simulink model "PhantomX_MK4"  (R2023a)
settings: Solver=FixedStepAuto  StartTime=0.0  StopTime=inf  FixedStep=0.00005  RelTol=1e-3
values from neighbouring files (symbols this model uses):
  angle_offsets_LF_RB = [45, 14.03624347, 60.58440117]    [InitialisationScript.m]    (also in simulation_setup.m)
  angle_offsets_middle = [0, 14.03624347, 60.58440117]    [InitialisationScript.m]    (also in simulation_setup.m)
  angle_offsets_RF_LB = [-45, 14.03624347, 60.58440117]    [InitialisationScript.m]    (also in simulation_setup.m)
  N = 16    [rl_setup.m]
  pid_D = 1    [InitialisationScript.m]    (also in simulation_setup.m)
  pid_filter_N = 100    [InitialisationScript.m]    (also in simulation_setup.m = 1000)
  pid_I = 0.2    [InitialisationScript.m]    (also in simulation_setup.m = 0.1)
  pid_P = 3    [InitialisationScript.m]    (also in simulation_setup.m = 600)
  x_offset = 0.2    [InitialisationScript.m]
  z_offset = -0.14    [InitialisationScript.m]
undefined symbols (not defined in the file or in its folder): LBL_sensory_data, left_side_torques, LFL_sensory_data, LML_sensory_data, RBL_sensory_data, RFL_sensory_data, right_side_torques, RML_sensory_data, X, Y, Z
libraries: sm_lib x30, slpidlib x18, Custom_Library x13, robotmaniplib x6, nesl_utility x3, rllib x1, simulink_extras x1
(part 1 of 4)
settings Model: SimulationMode=accelerator  PacingRate=0.089000  Creator=basti  LastModifiedBy=basti
settings SolverCC: EnableFixedStepZeroCrossing=on
settings ExplorerConfigSet: InternalSimMechanicsExplorerSettings="<ExplorerConfiguration><canonicalview>default</canonicalview><AnimationSetting><BasePlaybackSpeed>1.0</BasePlaybackSpeed><PlaybackSpeedFactor>1.0</PlaybackSpeedFactor></AnimationSetting><TilePanel><TileInfo><Tiles Columns=\"1\" Count=\"1\" Rows=\"1\"><Column Weight=\"1\"/><Row Weight=\"1\"/><Tile Height=\"1\" Width=\"1\" X=\"0\" Y=\"0\"/></Tiles></TileInfo><SceneInfo><SceneViewer><BGColor><R>0.800000011920928955</R><G>0.800000011920928955</G><B>0.800000011920928955</B></BGColor><Camera><DoPerspective>off</DoPerspective><Position><X>0.0139405011924200652</X><Y>-25.6990972548707113</Y><Z>0.0237848079060223108</Z></Position><Center><X>0.0139405011924200652</X><Y>8.89140117983633349e-07</Y><Z>0.0237848079060223108</Z></Center><Up><X>0</X><Y>-0</Y><Z>1</Z></Up><ViewLimDist>1</ViewLimDist><YLim>0.273259206556581868</YLim><XLim>0.411669828872019972</XLim></Camera></SceneViewer></SceneInfo></TilePanel><MechEditorPanel><Cameras/><GfxPanelCameraMap/><VideoCreator><PlaybackSpeedRatio>1.0</PlaybackSpeedRatio><FrameRate>60</FrameRate><VideoFormat>MPEG-4</VideoFormat><FrameSize>[1920 1080]</FrameSize></VideoCreator></MechEditorPanel></ExplorerConfiguration>"

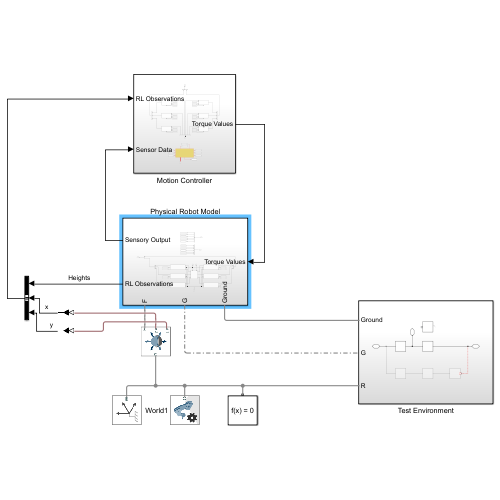
[thumbnail: Simulink's stored preview of the top-level diagram]
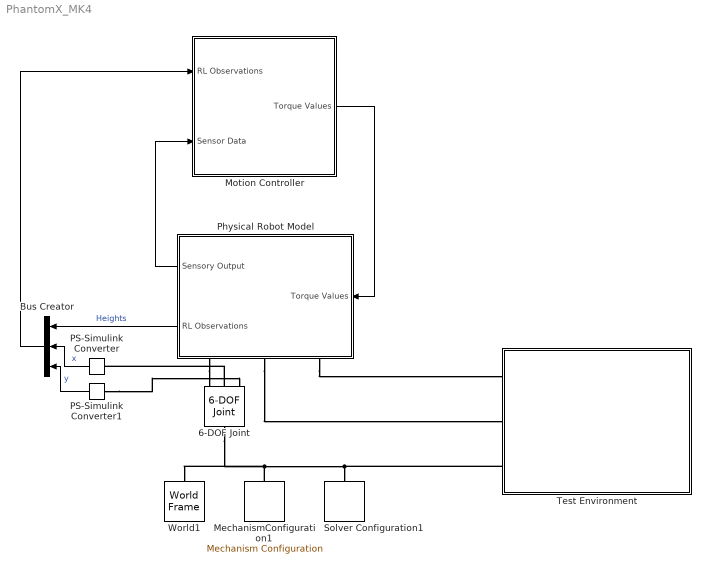
== system PhantomX_MK4 ==
  6-DOF Joint : sm_lib/Joints/6-DOF Joint  JointMode=Normal  SenseConstraintForce=off  SenseConstraintForceX=off  SenseConstraintForceY=off  SenseConstraintForceZ=off  SenseConstraintTorque=off  SenseConstraintTorqueX=off  SenseConstraintTorqueY=off  SenseConstraintTorqueZ=off  SenseTotalForce=off  SenseTotalForceX=off  SenseTotalForceY=off  SenseTotalForceZ=off  SenseTotalTorque=off  SenseTotalTorqueX=off  SenseTotalTorqueY=off  SenseTotalTorqueZ=off  CompositeWrenchDir=FollowerOnBase  CompositeWrenchFrame=BaseFrame  PxEquilibriumPosition=0  PxEquilibriumPositionUnits=m  PxSpringStiffness=0  PxSpringStiffnessUnits=N/m  PxDampingCoefficient=1e-8  PxDampingCoefficientUnits=N/(m/s)  PxTorqueActuationMode=NoTorque  PxMotionActuationMode=ComputedMotion  PxSensePosition=on  PxSenseVelocity=off  PxSenseAcceleration=off  PxSenseTorqueForce=off  PxSenseLowerLimitTorqueForce=off  PxSenseUpperLimitTorqueForce=off  PxLowerLimitSpecify=off  PxLowerLimitBound=-1  PxLowerLimitBoundUnits=m  PxLowerLimitStiffness=1e6  PxLowerLimitStiffnessUnits=N/m  PxLowerLimitDamping=1e3  PxLowerLimitDampingUnits=N/(m/s)  PxLowerLimitTransitionRegionWidth=1e-4  PxLowerLimitTransitionRegionWidthUnits=m  PxUpperLimitSpecify=off  PxUpperLimitBound=1  PxUpperLimitBoundUnits=m  PxUpperLimitStiffness=1e6  PxUpperLimitStiffnessUnits=N/m  PxUpperLimitDamping=1e3  PxUpperLimitDampingUnits=N/(m/s)  PxUpperLimitTransitionRegionWidth=1e-4  PxUpperLimitTransitionRegionWidthUnits=m  PxPositionTargetSpecify=off  PxPositionTargetPriority=High  PxPositionTargetValue=0  PxPositionTargetValueUnits=m  PxVelocityTargetSpecify=off  PxVelocityTargetPriority=High  PxVelocityTargetValue=0  PxVelocityTargetValueUnits=m/s  PyEquilibriumPosition=0  PyEquilibriumPositionUnits=m  PySpringStiffness=0  PySpringStiffnessUnits=N/m  PyDampingCoefficient=1e-8  PyDampingCoefficientUnits=N/(m/s)  PyTorqueActuationMode=NoTorque  PyMotionActuationMode=ComputedMotion  PySensePosition=on  PySenseVelocity=off  PySenseAcceleration=off  PySenseTorqueForce=off  PySenseLowerLimitTorqueForce=off  PySenseUpperLimitTorqueForce=off  PyLowerLimitSpecify=off  PyLowerLimitBound=-1  PyLowerLimitBoundUnits=m  PyLowerLimitStiffness=1e6  PyLowerLimitStiffnessUnits=N/m  PyLowerLimitDamping=1e3  PyLowerLimitDampingUnits=N/(m/s)  PyLowerLimitTransitionRegionWidth=1e-4  PyLowerLimitTransitionRegionWidthUnits=m  PyUpperLimitSpecify=off  PyUpperLimitBound=1  PyUpperLimitBoundUnits=m  PyUpperLimitStiffness=1e6  PyUpperLimitStiffnessUnits=N/m  PyUpperLimitDamping=1e3  PyUpperLimitDampingUnits=N/(m/s)  PyUpperLimitTransitionRegionWidth=1e-4  PyUpperLimitTransitionRegionWidthUnits=m  PyPositionTargetSpecify=off  PyPositionTargetPriority=High  PyPositionTargetValue=0  PyPositionTargetValueUnits=m  PyVelocityTargetSpecify=off  PyVelocityTargetPriority=High  PyVelocityTargetValue=0  PyVelocityTargetValueUnits=m/s  PzEquilibriumPosition=0  PzEquilibriumPositionUnits=m  PzSpringStiffness=0  PzSpringStiffnessUnits=N/m  PzDampingCoefficient=1e-8  PzDampingCoefficientUnits=N/(m/s)  PzTorqueActuationMode=NoTorque  PzMotionActuationMode=ComputedMotion  PzSensePosition=off  PzSenseVelocity=off  PzSenseAcceleration=off  PzSenseTorqueForce=off  PzSenseLowerLimitTorqueForce=off  PzSenseUpperLimitTorqueForce=off  PzLowerLimitSpecify=off  PzLowerLimitBound=-1  PzLowerLimitBoundUnits=m  PzLowerLimitStiffness=1e6  PzLowerLimitStiffnessUnits=N/m  PzLowerLimitDamping=1e3  PzLowerLimitDampingUnits=N/(m/s)  PzLowerLimitTransitionRegionWidth=1e-4  PzLowerLimitTransitionRegionWidthUnits=m  PzUpperLimitSpecify=off  PzUpperLimitBound=1  PzUpperLimitBoundUnits=m  PzUpperLimitStiffness=1e6  PzUpperLimitStiffnessUnits=N/m  PzUpperLimitDamping=1e3  PzUpperLimitDampingUnits=N/(m/s)  PzUpperLimitTransitionRegionWidth=1e-4  PzUpperLimitTransitionRegionWidthUnits=m  PzPositionTargetSpecify=off  PzPositionTargetPriority=High  PzPositionTargetValue=0  PzPositionTargetValueUnits=m  PzVelocityTargetSpecify=off  PzVelocityTargetPriority=High  PzVelocityTargetValue=0  PzVelocityTargetValueUnits=m/s  SphEqPosRotationMethod=None  SphEqPosRotationAngleUnits=deg  SphEqPosRotationStandardAxis=+Z  SphEqPosRotationAngle=0.0  SphEqPosRotationArbitraryAxis=[0 0 1]  SphEqPosFollAlignAxisA=+X  SphEqPosBaseAlignAxisA=+Y  SphEqPosFollAlignAxisB=+Y  SphEqPosBaseAlignAxisB=+Z  SphEqPosRotationSequenceAxes=FollowerAxes  SphEqPosRotationSequence=XYX  SphEqPosRotationSequenceAngles=[0 0 0]  SphEqPosRotationSequenceAnglesUnits=deg  SphEqPosRotationMatrix=[1 0 0; 0 1 0; 0 0 1]  SphEqPosQuaternion=[1 0 0 0]  SphSpringStiffness=0  SphSpringStiffnessUnits=N*m/deg  SphDampingCoefficient=0  SphDampingCoefficientUnits=N*m/(deg/s)  SphActuateTorqueX=off  SphActuateTorqueY=off  SphActuateTorqueZ=off  SphActuateTorque=off  SphTorqueActuationMode=NoTorque  SphMotionActuationMode=ComputedMotion  SphActuationFrame=BaseFrame  SphSensePosition=off  SphSenseVelocityX=off  SphSenseVelocityY=off  SphSenseVelocityZ=off  SphSenseVelocity=off  SphSenseAccelerationX=off  SphSenseAccelerationY=off  SphSenseAccelerationZ=off  SphSenseAcceleration=off  SphSenseTorqueX=off  SphSenseTorqueY=off  SphSenseTorqueZ=off  SphSenseTorqueForce=off  SphSenseLowerLimitTorqueMag=off  SphSenseUpperLimitTorqueMag=off  SphSensingFrame=BaseFrame  SphLowerLimitSpecify=off  SphLowerLimitBound=15  SphLowerLimitBoundUnits=deg  SphLowerLimitStiffness=1e4  SphLowerLimitStiffnessUnits=N*m/deg  SphLowerLimitDamping=10  SphLowerLimitDampingUnits=N*m/(deg/s)  SphLowerLimitTransitionRegionWidth=0.1  SphLowerLimitTransitionRegionWidthUnits=deg  SphUpperLimitSpecify=off  SphUpperLimitBound=45  SphUpperLimitBoundUnits=deg  SphUpperLimitStiffness=1e4  SphUpperLimitStiffnessUnits=N*m/deg  SphUpperLimitDamping=10  SphUpperLimitDampingUnits=N*m/(deg/s)  SphUpperLimitTransitionRegionWidth=0.1  SphUpperLimitTransitionRegionWidthUnits=deg  SphPositionTargetRotationMethod=None  SphPositionTargetRotationAngleUnits=deg  SphPositionTargetRotationStandardAxis=+Z  SphPositionTargetRotationAngle=0.0  SphPositionTargetRotationArbitraryAxis=[0 0 1]  SphPositionTargetFollAlignAxisA=+X  SphPositionTargetBaseAlignAxisA=+Y  SphPositionTargetFollAlignAxisB=+Y  SphPositionTargetBaseAlignAxisB=+Z  SphPositionTargetRotationSequenceAxes=FollowerAxes  SphPositionTargetRotationSequence=XYX  SphPositionTargetRotationSequenceAngles=[0 0 0]  SphPositionTargetRotationSequenceAnglesUnits=deg  SphPositionTargetRotationMatrix=[1 0 0; 0 1 0; 0 0 1]  SphPositionTargetQuaternion=[1 0 0 0]  SphPositionTargetSpecify=off  SphPositionTargetPriority=High  SphVelocityTargetValue=[0 0 0]  SphVelocityTargetValueUnits=deg/s  SphVelocityTargetSpecify=off  SphVelocityTargetPriority=High  SphVelocityTargetInFollowerFrame=on
  Bus Creator : BusCreator  Inputs=3
  MechanismConfiguration1 : sm_lib/Utilities/Mechanism Configuration  UniformGravity=Constant  GravityVector=gravity_vector  GravityVectorUnits=m/s^2  LinearizationDelta=1e-4  JointModeTransitionNonlinearIterations=4
  Motion Controller : Subsystem
  PS-Simulink Converter : nesl_utility/PS-Simulink Converter  PhysicalDomain=network_engine_domain  SubClassName=ps_output  LeftPortType=input  RightPortType=output  PseudoPeriodic=off  Frequencies=[]  VectorFormat=inherit  Unit=inherit  AffineConversion=off
  PS-Simulink Converter1 : nesl_utility/PS-Simulink Converter  PhysicalDomain=network_engine_domain  SubClassName=ps_output  LeftPortType=input  RightPortType=output  PseudoPeriodic=off  Frequencies=[]  VectorFormat=inherit  Unit=inherit  AffineConversion=off
  Physical Robot Model : Subsystem
      settings: PortSchema="{\"entries\":[{\"content\":{\"sides\":[{\"content\":{\"connectorIds\":[\"In1\"]},\"type\":\"ConnectorPlacement.EquallySpacedRectSide\",\"uuid\":\"88f2b8a6-de04-409c-a7b8-092446ee7a8a\"},{\"content\":{\"connectorIds\":[\"Out1\",\"Out2\"],\"side\":\"RIGHT\"},\"type\":\"ConnectorPlacement.EquallySpacedRectSide\",\"uuid\":\"05452a16-e9b5-441f-b64c-cc8b5f8bc9a9\"},{\"content\":{\"side\":\"TOP\"},\"type\":\"ConnectorPlacement.EquallySpacedRectSide\",\"uuid\":\"4b1c2960-246e-4fa9-be3c-7b063d456f3b\"},{\"content\":{\"connectorIds\":[\"RConn1\",\"RConn2\",\"RConn3\"],\"side\":\"BOTTOM\"},\"type\":\"ConnectorPlacement.EquallySpacedRectSide\",\"uuid\":\"877efe3a-863b-4f41-9fff-16e3adccfccc\"}]},\"type\":\"ConnectorPlacement.EquallySpacedConnector\",\"uuid\":\"79d07eaf-febf-441f-a139-eb85057738c3\"}],\"packageUris\":[\"http://schema.mathworks.com/mf0/Connector/R2020b\"],\"version\":\"1.0\"}"
  Solver Configuration1 : nesl_utility/Solver Configuration  PhysicalDomain=network_engine_domain  SubClassName=solver  LeftPortType=input  RightPortType=generic  Tones=[]  Harmonics=[]  SimulateNoise=off  Profile=off  UseLocalSampling=off  EnableSwitchedLinearOptims=on  FrequencyDomain=off  UseCCode=off  RelTol=0.001  AbsTol=0.001  MinStep=1e-09  ToWorkspace=off  RevertToSquareIcSolve=off  NumHomotopyIterations=100  PhasorMode=off  PhasorModeNumHarmonics=1  ConsistencySolver=NEWTON_XTOL_AFTER_FTOL  IndexReductionMethod=DerivativeReplacement  DoDC=off  ResidualTolerance=1e-09  ConsistencyTolSource=GLOBAL  ConsistencyAbsTol=0.001  ConsistencyRelTol=0.001  ConsistencyTolFactor=1e-4  UseLocalSolver=off  LocalSolverChoice=NE_BACKWARD_EULER_ADVANCER  ResolveIndetEquations=on  FunctionEvalNumThread=1  LocalSolverSampleTime=0.001  DoFixedCost=off  MaxNonlinIter=3  MaxModeIter=2  ComputeImpulses=off  ImpulseIterations=2  LinearAlgebra=Full  LinearAlgebraNumThread=0  EquationFormulation=NE_TIME_EF  DelaysMemoryBudget=2048  AutomaticFiltering=on  FilteringTimeConstant=0.001  PartitionStorageMethod=AS_NEEDED  PartitionMemoryBudget=1024  PartitionMethod=ROBUST
  Test Environment : Subsystem
  World1 : sm_lib/Frames and Transforms/World Frame
  wires:
  Physical Robot Model/1(Sensory Output) -> Motion Controller/2(Sensor Data)
  Motion Controller/1(Torque Values) -> Physical Robot Model/1(Torque Values)
  PS-Simulink Converter/1 -> Bus Creator/2  "x"
  Physical Robot Model/2(RL Observations) -> Bus Creator/1  "Heights"
  Bus Creator/1 -> Motion Controller/1(RL Observations)
  PS-Simulink Converter1/1 -> Bus Creator/3  "y"
  connections:
  MechanismConfiguration1/RConn1 -- World1/RConn1 -- 6-DOF Joint/LConn1 -- Test Environment/LConn3 -- Solver Configuration1/RConn1
  Physical Robot Model/RConn2 -- Test Environment/LConn2
  Physical Robot Model/RConn3 -- 6-DOF Joint/RConn1
  Physical Robot Model/RConn1 -- Test Environment/LConn1
  6-DOF Joint/RConn2 -- PS-Simulink Converter/LConn1
  PS-Simulink Converter1/LConn1 -- 6-DOF Joint/RConn3

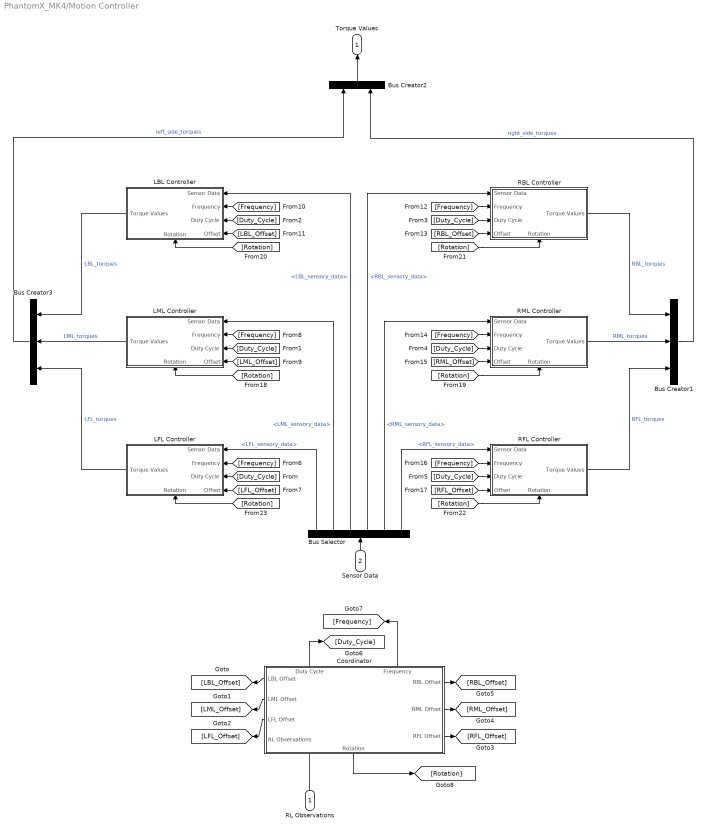
== system PhantomX_MK4/Motion Controller ==
  RL Observations : Inport
  Sensor Data : Inport  Port=2
  Bus Creator1 : BusCreator  Inputs=3
  Bus Creator2 : BusCreator  Inputs=left_side_torques,right_side_torques
  Bus Creator3 : BusCreator  Inputs=3
  Bus Selector : BusSelector  OutputSignals=LFL_sensory_data,LML_sensory_data,LBL_sensory_data,RBL_sensory_data,RML_sensory_data,RFL_sensory_data
  Coordinator : Subsystem
      settings: PortSchema="{\"entries\":[{\"content\":{\"sides\":[{\"content\":{\"connectorIds\":[\"Out7\",\"Out8\",\"Out9\",\"In1\"]},\"type\":\"ConnectorPlacement.EquallySpacedRectSide\",\"uuid\":\"0589587c-a667-4b39-9acd-4e49c48a2b81\"},{\"content\":{\"connectorIds\":[\"Out1\",\"Out2\",\"Out3\"],\"side\":\"RIGHT\"},\"type\":\"ConnectorPlacement.EquallySpacedRectSide\",\"uuid\":\"38142eef-ff42-4a7a-ad69-e4b368cabc10\"},{\"content\":{\"connectorIds\":[\"Out5\",\"Out6\"],\"side\":\"TOP\"},\"type\":\"ConnectorPlacement.EquallySpacedRectSide\",\"uuid\":\"0cab318c-da30-4070-96db-6d2791547378\"},{\"content\":{\"connectorIds\":[\"Out4\"],\"side\":\"BOTTOM\"},\"type\":\"ConnectorPlacement.EquallySpacedRectSide\",\"uuid\":\"5a744909-6628-4943-920b-0f55011947f4\"}]},\"type\":\"ConnectorPlacement.EquallySpacedConnector\",\"uuid\":\"f4523b82-4d9f-456b-8594-48e9d89b7aea\"}],\"packageUris\":[\"http://schema.mathworks.com/mf0/Connector/R2020b\"],\"version\":\"1.0\"}"
  LBL Controller : Subsystem
      settings: PortSchema="{\"entries\":[{\"content\":{\"sides\":[{\"content\":{\"connectorIds\":[\"In1\",\"In2\",\"In3\",\"In4\"]},\"type\":\"ConnectorPlacement.EquallySpacedRectSide\",\"uuid\":\"61807659-790a-4fcc-8eea-bb1747959d2c\"},{\"content\":{\"connectorIds\":[\"Out1\"],\"side\":\"RIGHT\"},\"type\":\"ConnectorPlacement.EquallySpacedRectSide\",\"uuid\":\"beab48f8-df50-4720-a4fe-1084d91255e1\"},{\"content\":{\"side\":\"TOP\"},\"type\":\"ConnectorPlacement.EquallySpacedRectSide\",\"uuid\":\"df2f0e11-b286-4413-8948-937711258f59\"},{\"content\":{\"connectorIds\":[\"In5\"],\"side\":\"BOTTOM\"},\"type\":\"ConnectorPlacement.EquallySpacedRectSide\",\"uuid\":\"177fd513-fdd6-4ae0-8805-86acc5cb073f\"}]},\"type\":\"ConnectorPlacement.EquallySpacedConnector\",\"uuid\":\"735c34ff-c8fb-4d96-b4d8-f985913f524f\"}],\"packageUris\":[\"http://schema.mathworks.com/mf0/Connector/R2020b\"],\"version\":\"1.0\"}"
  LFL Controller : Subsystem
      settings: PortSchema="{\"entries\":[{\"content\":{\"sides\":[{\"content\":{\"connectorIds\":[\"In1\",\"In2\",\"In3\",\"In4\"]},\"type\":\"ConnectorPlacement.EquallySpacedRectSide\",\"uuid\":\"61807659-790a-4fcc-8eea-bb1747959d2c\"},{\"content\":{\"connectorIds\":[\"Out1\"],\"side\":\"RIGHT\"},\"type\":\"ConnectorPlacement.EquallySpacedRectSide\",\"uuid\":\"beab48f8-df50-4720-a4fe-1084d91255e1\"},{\"content\":{\"side\":\"TOP\"},\"type\":\"ConnectorPlacement.EquallySpacedRectSide\",\"uuid\":\"df2f0e11-b286-4413-8948-937711258f59\"},{\"content\":{\"connectorIds\":[\"In5\"],\"side\":\"BOTTOM\"},\"type\":\"ConnectorPlacement.EquallySpacedRectSide\",\"uuid\":\"f745b799-b20b-4ee3-af3a-7f9c6b228ef2\"}]},\"type\":\"ConnectorPlacement.EquallySpacedConnector\",\"uuid\":\"735c34ff-c8fb-4d96-b4d8-f985913f524f\"}],\"packageUris\":[\"http://schema.mathworks.com/mf0/Connector/R2020b\"],\"version\":\"1.0\"}"
  LML Controller : Subsystem
      settings: PortSchema="{\"entries\":[{\"content\":{\"sides\":[{\"content\":{\"connectorIds\":[\"In1\",\"In2\",\"In3\",\"In4\"]},\"type\":\"ConnectorPlacement.EquallySpacedRectSide\",\"uuid\":\"61807659-790a-4fcc-8eea-bb1747959d2c\"},{\"content\":{\"connectorIds\":[\"Out1\"],\"side\":\"RIGHT\"},\"type\":\"ConnectorPlacement.EquallySpacedRectSide\",\"uuid\":\"beab48f8-df50-4720-a4fe-1084d91255e1\"},{\"content\":{\"side\":\"TOP\"},\"type\":\"ConnectorPlacement.EquallySpacedRectSide\",\"uuid\":\"df2f0e11-b286-4413-8948-937711258f59\"},{\"content\":{\"connectorIds\":[\"In5\"],\"side\":\"BOTTOM\"},\"type\":\"ConnectorPlacement.EquallySpacedRectSide\",\"uuid\":\"b53235e4-d895-4a2a-8595-c01fb6c9295f\"}]},\"type\":\"ConnectorPlacement.EquallySpacedConnector\",\"uuid\":\"735c34ff-c8fb-4d96-b4d8-f985913f524f\"}],\"packageUris\":[\"http://schema.mathworks.com/mf0/Connector/R2020b\"],\"version\":\"1.0\"}"
  RBL Controller : Subsystem
      settings: PortSchema="{\"entries\":[{\"content\":{\"sides\":[{\"content\":{\"connectorIds\":[\"In1\",\"In2\",\"In3\",\"In4\"]},\"type\":\"ConnectorPlacement.EquallySpacedRectSide\",\"uuid\":\"61807659-790a-4fcc-8eea-bb1747959d2c\"},{\"content\":{\"connectorIds\":[\"Out1\"],\"side\":\"RIGHT\"},\"type\":\"ConnectorPlacement.EquallySpacedRectSide\",\"uuid\":\"beab48f8-df50-4720-a4fe-1084d91255e1\"},{\"content\":{\"side\":\"TOP\"},\"type\":\"ConnectorPlacement.EquallySpacedRectSide\",\"uuid\":\"df2f0e11-b286-4413-8948-937711258f59\"},{\"content\":{\"connectorIds\":[\"In5\"],\"side\":\"BOTTOM\"},\"type\":\"ConnectorPlacement.EquallySpacedRectSide\",\"uuid\":\"541f6a39-2cd2-4849-82a6-ba8e08840f40\"}]},\"type\":\"ConnectorPlacement.EquallySpacedConnector\",\"uuid\":\"735c34ff-c8fb-4d96-b4d8-f985913f524f\"}],\"packageUris\":[\"http://schema.mathworks.com/mf0/Connector/R2020b\"],\"version\":\"1.0\"}"
  RFL Controller : Subsystem
      settings: PortSchema="{\"entries\":[{\"content\":{\"sides\":[{\"content\":{\"connectorIds\":[\"In1\",\"In2\",\"In3\",\"In4\"]},\"type\":\"ConnectorPlacement.EquallySpacedRectSide\",\"uuid\":\"e919d3cb-cb22-4ae7-9921-75070e82dfc0\"},{\"content\":{\"connectorIds\":[\"Out1\"],\"side\":\"RIGHT\"},\"type\":\"ConnectorPlacement.EquallySpacedRectSide\",\"uuid\":\"1bac186a-4e1d-4bd0-8d36-9d7d141f01e6\"},{\"content\":{\"side\":\"TOP\"},\"type\":\"ConnectorPlacement.EquallySpacedRectSide\",\"uuid\":\"779ab6f5-6e15-4076-9acb-2bf4234ddf49\"},{\"content\":{\"connectorIds\":[\"In5\"],\"side\":\"BOTTOM\"},\"type\":\"ConnectorPlacement.EquallySpacedRectSide\",\"uuid\":\"a3aab620-5d97-425b-8a2a-088ff14d55a6\"}]},\"type\":\"ConnectorPlacement.EquallySpacedConnector\",\"uuid\":\"b8d6bd7a-da61-4133-9438-dd2459d5cc9a\"}],\"packageUris\":[\"http://schema.mathworks.com/mf0/Connector/R2020b\"],\"version\":\"1.0\"}"
  RML Controller : Subsystem
      settings: PortSchema="{\"entries\":[{\"content\":{\"sides\":[{\"content\":{\"connectorIds\":[\"In1\",\"In2\",\"In3\",\"In4\"]},\"type\":\"ConnectorPlacement.EquallySpacedRectSide\",\"uuid\":\"61807659-790a-4fcc-8eea-bb1747959d2c\"},{\"content\":{\"connectorIds\":[\"Out1\"],\"side\":\"RIGHT\"},\"type\":\"ConnectorPlacement.EquallySpacedRectSide\",\"uuid\":\"beab48f8-df50-4720-a4fe-1084d91255e1\"},{\"content\":{\"side\":\"TOP\"},\"type\":\"ConnectorPlacement.EquallySpacedRectSide\",\"uuid\":\"df2f0e11-b286-4413-8948-937711258f59\"},{\"content\":{\"connectorIds\":[\"In5\"],\"side\":\"BOTTOM\"},\"type\":\"ConnectorPlacement.EquallySpacedRectSide\",\"uuid\":\"7df11b11-4116-490c-abf6-aeb9f4bc13f8\"}]},\"type\":\"ConnectorPlacement.EquallySpacedConnector\",\"uuid\":\"735c34ff-c8fb-4d96-b4d8-f985913f524f\"}],\"packageUris\":[\"http://schema.mathworks.com/mf0/Connector/R2020b\"],\"version\":\"1.0\"}"
  Torque Values : Outport
  wires:
  Sensor Data/1 -> Bus Selector/1
  Bus Creator2/1 -> Torque Values/1
  Bus Creator1/1 -> Bus Creator2/2  "right_side_torques"
  Bus Creator3/1 -> Bus Creator2/1  "left_side_torques"
  LFL Controller/1(Torque Values) -> Bus Creator3/3  "LFL_torques"
  LML Controller/1(Torque Values) -> Bus Creator3/2  "LML_torques"
  LBL Controller/1(Torque Values) -> Bus Creator3/1  "LBL_torques"
  RBL Controller/1(Torque Values) -> Bus Creator1/1  "RBL_torques"
  RML Controller/1(Torque Values) -> Bus Creator1/2  "RML_torques"
  RFL Controller/1(Torque Values) -> Bus Creator1/3  "RFL_torques"
  Coordinator/7(LBL Offset) -> [LBL_Offset]
  Coordinator/8(LML Offset) -> [LML_Offset]
  Coordinator/9(LFL Offset) -> [LFL_Offset]
  Coordinator/3(RFL Offset) -> [RFL_Offset]
  Coordinator/2(RML Offset) -> [RML_Offset]
  Coordinator/1(RBL Offset) -> [RBL_Offset]
  Coordinator/5(Duty Cycle) -> [Duty_Cycle]
  Coordinator/6(Frequency) -> [Frequency]
  [Duty_Cycle] -> LFL Controller/3(Duty Cycle)
  [Duty_Cycle] -> LML Controller/3(Duty Cycle)
  [Duty_Cycle] -> LBL Controller/3(Duty Cycle)
  [Duty_Cycle] -> RBL Controller/3(Duty Cycle)
  [Duty_Cycle] -> RML Controller/3(Duty Cycle)
  [Duty_Cycle] -> RFL Controller/3(Duty Cycle)
  [Frequency] -> LFL Controller/2(Frequency)
  [LFL_Offset] -> LFL Controller/4(Offset)
  [LML_Offset] -> LML Controller/4(Offset)
  [Frequency] -> LML Controller/2(Frequency)
  [LBL_Offset] -> LBL Controller/4(Offset)
  [Frequency] -> LBL Controller/2(Frequency)
  [Frequency] -> RBL Controller/2(Frequency)
  [RBL_Offset] -> RBL Controller/4(Offset)
  [RML_Offset] -> RML Controller/4(Offset)
  [Frequency] -> RML Controller/2(Frequency)
  [Frequency] -> RFL Controller/2(Frequency)
  [RFL_Offset] -> RFL Controller/4(Offset)
  Bus Selector/4 -> RBL Controller/1(Sensor Data)  "<RBL_sensory_data>"
  Bus Selector/1 -> LFL Controller/1(Sensor Data)  "<LFL_sensory_data>"
  Bus Selector/2 -> LML Controller/1(Sensor Data)  "<LML_sensory_data>"
  Bus Selector/5 -> RML Controller/1(Sensor Data)  "<RML_sensory_data>"
  Bus Selector/3 -> LBL Controller/1(Sensor Data)  "<LBL_sensory_data>"
  Bus Selector/6 -> RFL Controller/1(Sensor Data)  "<RFL_sensory_data>"
  [Rotation] -> LML Controller/5(Rotation)
  Coordinator/4(Rotation) -> [Rotation]
  [Rotation] -> RML Controller/5(Rotation)
  [Rotation] -> LBL Controller/5(Rotation)
  [Rotation] -> RBL Controller/5(Rotation)
  [Rotation] -> LFL Controller/5(Rotation)
  [Rotation] -> RFL Controller/5(Rotation)
  RL Observations/1 -> ?

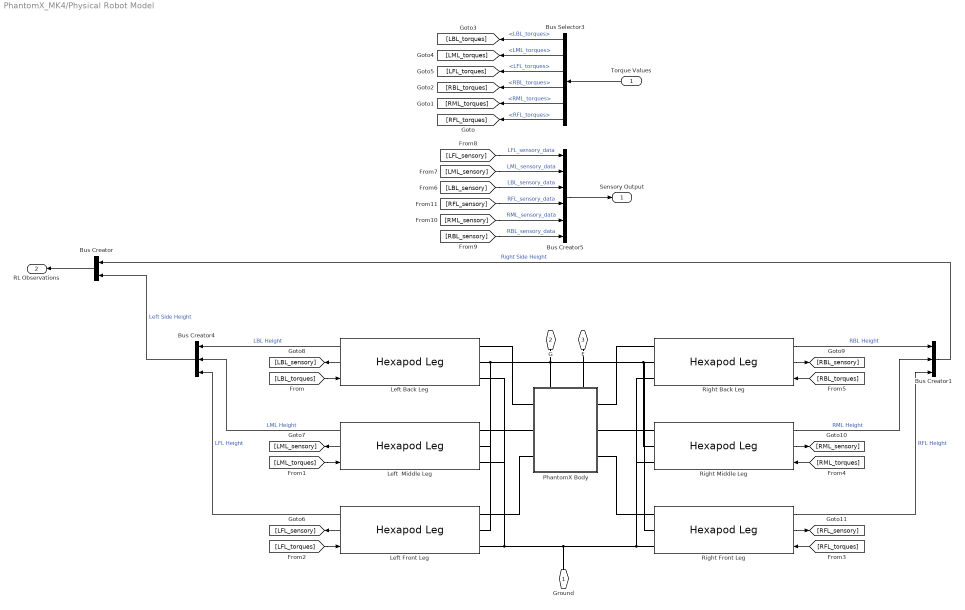
== system PhantomX_MK4/Physical Robot Model ==
  Torque Values : Inport
  Bus Creator : BusCreator  Inputs=2
  Bus Creator1 : BusCreator  Inputs=3
  Bus Creator4 : BusCreator  Inputs=3
  Bus Creator5 : BusCreator  Inputs=LFL_sensory_data,LML_sensory_data,LBL_sensory_data,RFL_sensory_data,RML_sensory_data,RBL_sensory_data
  Bus Selector3 : BusSelector  OutputSignals=left_side_torques.LBL_torques,left_side_torques.LML_torques,left_side_torques.LFL_torques,right_side_torques.RBL_torques,right_side_torques.RML_torques,right_side_torques.RFL_torques
  Left  Middle Leg : Custom_Library/Hexapod Leg  SystemSampleTime=-1  VariantActivationTime=update diagram  Latency=0  AutoFrameSizeCalculation=off
      settings: SourceProductName=Custom Hexapod Blocks  PortSchema="{\"entries\":[{\"content\":{\"sides\":[{\"content\":{\"connectorIds\":[\"LConn1\",\"LConn2\",\"LConn3\"]},\"type\":\"ConnectorPlacement.EquallySpacedRectSide\",\"uuid\":\"f49879d6-ba76-4ec0-9cde-e27e7d64cb43\"},{\"content\":{\"connectorIds\":[\"In1\",\"Out1\",\"Out2\"],\"side\":\"RIGHT\"},\"type\":\"ConnectorPlacement.EquallySpacedRectSide\",\"uuid\":\"65b15dde-e5d7-47cb-8ac1-e9e029e05721\"},{\"content\":{\"side\":\"TOP\"},\"type\":\"ConnectorPlacement.EquallySpacedRectSide\",\"uuid\":\"11559e5b-a1be-4233-aeb2-21e170c4e963\"}]},\"type\":\"ConnectorPlacement.EquallySpacedConnector\",\"uuid\":\"c4377ad5-9946-4ac5-9145-d9e25f76b3b4\"}],\"packageUris\":[\"http://schema.mathworks.com/mf0/Connector/R2020b\"],\"version\":\"1.0\"}"
  Left Back Leg : Custom_Library/Hexapod Leg  SystemSampleTime=-1  VariantActivationTime=update diagram  Latency=0  AutoFrameSizeCalculation=off
      settings: SourceProductName=Custom Hexapod Blocks  PortSchema="{\"entries\":[{\"content\":{\"sides\":[{\"content\":{\"connectorIds\":[\"LConn1\",\"LConn2\",\"LConn3\"]},\"type\":\"ConnectorPlacement.EquallySpacedRectSide\",\"uuid\":\"f49879d6-ba76-4ec0-9cde-e27e7d64cb43\"},{\"content\":{\"connectorIds\":[\"In1\",\"Out1\",\"Out2\"],\"side\":\"RIGHT\"},\"type\":\"ConnectorPlacement.EquallySpacedRectSide\",\"uuid\":\"65b15dde-e5d7-47cb-8ac1-e9e029e05721\"},{\"content\":{\"side\":\"TOP\"},\"type\":\"ConnectorPlacement.EquallySpacedRectSide\",\"uuid\":\"11559e5b-a1be-4233-aeb2-21e170c4e963\"}]},\"type\":\"ConnectorPlacement.EquallySpacedConnector\",\"uuid\":\"c4377ad5-9946-4ac5-9145-d9e25f76b3b4\"}],\"packageUris\":[\"http://schema.mathworks.com/mf0/Connector/R2020b\"],\"version\":\"1.0\"}"
  Left Front Leg : Custom_Library/Hexapod Leg  SystemSampleTime=-1  VariantActivationTime=update diagram  Latency=0  AutoFrameSizeCalculation=off
      settings: SourceProductName=Custom Hexapod Blocks  PortSchema="{\"entries\":[{\"content\":{\"sides\":[{\"content\":{\"connectorIds\":[\"LConn1\",\"LConn2\",\"LConn3\"]},\"type\":\"ConnectorPlacement.EquallySpacedRectSide\",\"uuid\":\"f49879d6-ba76-4ec0-9cde-e27e7d64cb43\"},{\"content\":{\"connectorIds\":[\"In1\",\"Out1\",\"Out2\"],\"side\":\"RIGHT\"},\"type\":\"ConnectorPlacement.EquallySpacedRectSide\",\"uuid\":\"65b15dde-e5d7-47cb-8ac1-e9e029e05721\"},{\"content\":{\"side\":\"TOP\"},\"type\":\"ConnectorPlacement.EquallySpacedRectSide\",\"uuid\":\"11559e5b-a1be-4233-aeb2-21e170c4e963\"}]},\"type\":\"ConnectorPlacement.EquallySpacedConnector\",\"uuid\":\"c4377ad5-9946-4ac5-9145-d9e25f76b3b4\"}],\"packageUris\":[\"http://schema.mathworks.com/mf0/Connector/R2020b\"],\"version\":\"1.0\"}"
  PhantomX Body : Subsystem
      settings: PortSchema="{\"entries\":[{\"content\":{\"sides\":[{\"content\":{\"connectorIds\":[\"LConn1\",\"LConn2\",\"LConn3\"]},\"type\":\"ConnectorPlacement.EquallySpacedRectSide\",\"uuid\":\"45e61c57-2f9a-4e87-9f4b-cbd725790b51\"},{\"content\":{\"connectorIds\":[\"RConn1\",\"RConn2\",\"RConn3\"],\"side\":\"RIGHT\"},\"type\":\"ConnectorPlacement.EquallySpacedRectSide\",\"uuid\":\"eaad478e-8ea6-4d0b-92b6-9d97b6898032\"},{\"content\":{\"connectorIds\":[\"LConn4\",\"LConn5\"],\"side\":\"TOP\"},\"type\":\"ConnectorPlacement.EquallySpacedRectSide\",\"uuid\":\"114e3ca6-7741-46e1-b6ae-33cac0b6bb49\"},{\"content\":{\"side\":\"BOTTOM\"},\"type\":\"ConnectorPlacement.EquallySpacedRectSide\",\"uuid\":\"86f8f33e-67eb-48f1-9000-f1c4835d1932\"}]},\"type\":\"ConnectorPlacement.EquallySpacedConnector\",\"uuid\":\"a9826fe9-ed84-48b9-b774-649deb3d7c78\"}],\"packageUris\":[\"http://schema.mathworks.com/mf0/Connector/R2020b\"],\"version\":\"1.0\"}"
  Right Back Leg : Custom_Library/Hexapod Leg  SystemSampleTime=-1  VariantActivationTime=update diagram  Latency=0  AutoFrameSizeCalculation=off
      settings: SourceProductName=Custom Hexapod Blocks  PortSchema="{\"entries\":[{\"content\":{\"sides\":[{\"content\":{\"connectorIds\":[\"LConn1\",\"LConn2\",\"LConn3\"]},\"type\":\"ConnectorPlacement.EquallySpacedRectSide\",\"uuid\":\"f49879d6-ba76-4ec0-9cde-e27e7d64cb43\"},{\"content\":{\"connectorIds\":[\"In1\",\"Out1\",\"Out2\"],\"side\":\"RIGHT\"},\"type\":\"ConnectorPlacement.EquallySpacedRectSide\",\"uuid\":\"65b15dde-e5d7-47cb-8ac1-e9e029e05721\"},{\"content\":{\"side\":\"TOP\"},\"type\":\"ConnectorPlacement.EquallySpacedRectSide\",\"uuid\":\"11559e5b-a1be-4233-aeb2-21e170c4e963\"}]},\"type\":\"ConnectorPlacement.EquallySpacedConnector\",\"uuid\":\"c4377ad5-9946-4ac5-9145-d9e25f76b3b4\"}],\"packageUris\":[\"http://schema.mathworks.com/mf0/Connector/R2020b\"],\"version\":\"1.0\"}"
  Right Front Leg : Custom_Library/Hexapod Leg  SystemSampleTime=-1  VariantActivationTime=update diagram  Latency=0  AutoFrameSizeCalculation=off
      settings: SourceProductName=Custom Hexapod Blocks  PortSchema="{\"entries\":[{\"content\":{\"sides\":[{\"content\":{\"connectorIds\":[\"LConn1\",\"LConn2\",\"LConn3\"]},\"type\":\"ConnectorPlacement.EquallySpacedRectSide\",\"uuid\":\"f49879d6-ba76-4ec0-9cde-e27e7d64cb43\"},{\"content\":{\"connectorIds\":[\"In1\",\"Out1\",\"Out2\"],\"side\":\"RIGHT\"},\"type\":\"ConnectorPlacement.EquallySpacedRectSide\",\"uuid\":\"65b15dde-e5d7-47cb-8ac1-e9e029e05721\"},{\"content\":{\"side\":\"TOP\"},\"type\":\"ConnectorPlacement.EquallySpacedRectSide\",\"uuid\":\"11559e5b-a1be-4233-aeb2-21e170c4e963\"}]},\"type\":\"ConnectorPlacement.EquallySpacedConnector\",\"uuid\":\"c4377ad5-9946-4ac5-9145-d9e25f76b3b4\"}],\"packageUris\":[\"http://schema.mathworks.com/mf0/Connector/R2020b\"],\"version\":\"1.0\"}"
  Right Middle Leg : Custom_Library/Hexapod Leg  SystemSampleTime=-1  VariantActivationTime=update diagram  Latency=0  AutoFrameSizeCalculation=off
      settings: SourceProductName=Custom Hexapod Blocks  PortSchema="{\"entries\":[{\"content\":{\"sides\":[{\"content\":{\"connectorIds\":[\"LConn1\",\"LConn2\",\"LConn3\"]},\"type\":\"ConnectorPlacement.EquallySpacedRectSide\",\"uuid\":\"f49879d6-ba76-4ec0-9cde-e27e7d64cb43\"},{\"content\":{\"connectorIds\":[\"In1\",\"Out1\",\"Out2\"],\"side\":\"RIGHT\"},\"type\":\"ConnectorPlacement.EquallySpacedRectSide\",\"uuid\":\"65b15dde-e5d7-47cb-8ac1-e9e029e05721\"},{\"content\":{\"side\":\"TOP\"},\"type\":\"ConnectorPlacement.EquallySpacedRectSide\",\"uuid\":\"11559e5b-a1be-4233-aeb2-21e170c4e963\"}]},\"type\":\"ConnectorPlacement.EquallySpacedConnector\",\"uuid\":\"c4377ad5-9946-4ac5-9145-d9e25f76b3b4\"}],\"packageUris\":[\"http://schema.mathworks.com/mf0/Connector/R2020b\"],\"version\":\"1.0\"}"
  Ground : PMIOPort  Side=Right
  G : PMIOPort  Port=2  Side=Right
  F : PMIOPort  Port=3  Side=Right
  Sensory Output : Outport
  RL Observations : Outport  Port=2
  wires:
  Left Front Leg/1 -> [LFL_sensory]
  Torque Values/1 -> Bus Selector3/1
  Bus Creator/1 -> RL Observations/1
  Bus Creator4/1 -> Bus Creator/2  "Left Side Height"
  [LBL_torques] -> Left Back Leg/1
  [LML_torques] -> Left  Middle Leg/1
  [LFL_torques] -> Left Front Leg/1
  Left  Middle Leg/1 -> [LML_sensory]
  Left Back Leg/1 -> [LBL_sensory]
  Right Back Leg/1 -> [RBL_sensory]
  Right Middle Leg/1 -> [RML_sensory]
  Right Front Leg/1 -> [RFL_sensory]
  [RFL_torques] -> Right Front Leg/1
  [RML_torques] -> Right Middle Leg/1
  [RBL_torques] -> Right Back Leg/1
  Bus Creator5/1 -> Sensory Output/1
  [LFL_sensory] -> Bus Creator5/1  "LFL_sensory_data"
  [LML_sensory] -> Bus Creator5/2  "LML_sensory_data"
  [LBL_sensory] -> Bus Creator5/3  "LBL_sensory_data"
  [RFL_sensory] -> Bus Creator5/4  "RFL_sensory_data"
  [RML_sensory] -> Bus Creator5/5  "RML_sensory_data"
  [RBL_sensory] -> Bus Creator5/6  "RBL_sensory_data"
  Bus Selector3/1 -> [LBL_torques]  "<LBL_torques>"
  Bus Selector3/2 -> [LML_torques]  "<LML_torques>"
  Bus Selector3/3 -> [LFL_torques]  "<LFL_torques>"
  Bus Selector3/4 -> [RBL_torques]  "<RBL_torques>"
  Bus Selector3/5 -> [RML_torques]  "<RML_torques>"
  Bus Selector3/6 -> [RFL_torques]  "<RFL_torques>"
  Left  Middle Leg/2 -> Bus Creator4/2  "LML Height"
  Left Back Leg/2 -> Bus Creator4/1  "LBL Height"
  Left Front Leg/2 -> Bus Creator4/3  "LFL Height"
  Right Back Leg/2 -> Bus Creator1/1  "RBL Height"
  Right Middle Leg/2 -> Bus Creator1/2  "RML Height"
  Right Front Leg/2 -> Bus Creator1/3  "RFL Height"
  Bus Creator1/1 -> Bus Creator/1  "Right Side Height"
  connections:
  PhantomX Body/LConn5 -- F/RConn1
  Left Front Leg/LConn3 -- PhantomX Body/LConn3
  Ground/RConn1 -- Right Front Leg/LConn1 -- Right Middle Leg/LConn1 -- Right Back Leg/LConn1 -- Left Front Leg/LConn1 -- Left  Middle Leg/LConn1 -- Left Back Leg/LConn1
  Left Back Leg/LConn3 -- PhantomX Body/LConn1
  Left  Middle Leg/LConn3 -- PhantomX Body/LConn2
  G/RConn1 -- Right Front Leg/LConn2 -- Right Middle Leg/LConn2 -- Right Back Leg/LConn2 -- PhantomX Body/LConn4 -- Left Back Leg/LConn2 -- Left Front Leg/LConn2 -- Left  Middle Leg/LConn2
  Right Middle Leg/LConn3 -- PhantomX Body/RConn2
  Right Front Leg/LConn3 -- PhantomX Body/RConn3
  Right Back Leg/LConn3 -- PhantomX Body/RConn1

== system PhantomX_MK4/Test Environment ==
  Brick Solid : sm_lib/Body Elements/Brick Solid  GraphicAmbientColor=[0.15 0.15 0.15 1.0]  BasedOnType=Density  BrickDimensions=[50 10 0.1]  BrickDimensionsUnits=m  CenterOfMass=[0 0 0]  CenterOfMassUnits=m  GraphicDiffuseColor=[0.6 0.8 1.0]  Density=1000  DensityUnits=kg/m^3  DoExposeReferenceFrame=on  GraphicEmissiveColor=[0.0 0.0 0.0 1.0]  ExportEntireGeometry=on  SerializedFrames=<Frames/>  MarkerShape=Sphere  MarkerSize=10  GraphicType=FromGeometry  InertiaType=CalculateFromGeometry  Mass=1  MassUnits=kg  MomentsOfInertia=[1 1 1]  MomentsOfInertiaUnits=kg*m^2  GraphicOpacity=1.0  ProductsOfInertia=[0 0 0]  ProductsOfInertiaUnits=kg*m^2  GraphicShininess=75  GraphicSpecularColor=[0.5 0.5 0.5 1.0]  GraphicVisPropType=SimpleVisualProperties
  Brick Solid1 : sm_lib/Body Elements/Brick Solid  Commented=on  GraphicAmbientColor=[0.15 0.15 0.15 1.0]  BasedOnType=Density  BrickDimensions=[10 10 0.1]  BrickDimensionsUnits=m  CenterOfMass=[0 0 0]  CenterOfMassUnits=m  GraphicDiffuseColor=[0.6 0.8 1.0]  Density=1000  DensityUnits=kg/m^3  DoExposeReferenceFrame=on  GraphicEmissiveColor=[0.0 0.0 0.0 1.0]  ExportEntireGeometry=on  SerializedFrames=<Frames/>  MarkerShape=Sphere  MarkerSize=10  GraphicType=FromGeometry  InertiaType=CalculateFromGeometry  Mass=1  MassUnits=kg  MomentsOfInertia=[1 1 1]  MomentsOfInertiaUnits=kg*m^2  GraphicOpacity=1.0  ProductsOfInertia=[0 0 0]  ProductsOfInertiaUnits=kg*m^2  GraphicShininess=75  GraphicSpecularColor=[0.5 0.5 0.5 1.0]  GraphicVisPropType=SimpleVisualProperties
  Infinite Plane : sm_lib/Curves and Surfaces/Infinite Plane  GraphicType=Rectangle  GraphicPlaneWidth=1  GraphicPlaneWidthUnits=m  GraphicPlaneHeight=1  GraphicPlaneHeightUnits=m  GraphicVisPropType=SimpleVisualProperties  GraphicDiffuseColor=[0.5 0.5 0.5]  GraphicOpacity=0.25  GraphicSpecularColor=[0.5 0.5 0.5 1.0]  GraphicAmbientColor=[0.15 0.15 0.15 1.0]  GraphicEmissiveColor=[0.0 0.0 0.0 1.0]  GraphicShininess=75
  Rotation : sm_lib/Frames and Transforms/Rigid Transform  Commented=on  TranslationMethod=None  TranslationStandardOffset=plane_offset  TranslationStandardOffsetUnits=m  TranslationStandardAxis=-Z  TranslationCartesianOffset=[0 0 0]  TranslationCartesianOffsetUnits=m  TranslationROffset=0  TranslationROffsetUnits=m  TranslationZOffset=0  TranslationZOffsetUnits=m  TranslationThetaOffset=0  TranslationThetaOffsetUnits=deg  RotationMethod=StandardAxis  RotationAngleUnits=deg  RotationStandardAxis=+Y  RotationAngle=-5  RotationArbitraryAxis=[0 0 1]  FollAlignAxisA=+X  BaseAlignAxisA=+Y  FollAlignAxisB=+Y  BaseAlignAxisB=+Z  RotationSequenceAxes=FollowerAxes  RotationSequence=XYX  RotationSequenceAngles=[0 0 0]  RotationSequenceAnglesUnits=deg  RotationMatrix=[1 0 0; 0 1 0; 0 0 1]  Quaternion=[1 0 0 0]
  Translation : sm_lib/Frames and Transforms/Rigid Transform  Commented=on  TranslationMethod=StandardAxis  TranslationStandardOffset=3  TranslationStandardOffsetUnits=m  TranslationStandardAxis=+X  TranslationCartesianOffset=[0 0 0]  TranslationCartesianOffsetUnits=m  TranslationROffset=0  TranslationROffsetUnits=m  TranslationZOffset=0  TranslationZOffsetUnits=m  TranslationThetaOffset=0  TranslationThetaOffsetUnits=deg  RotationMethod=None  RotationAngleUnits=deg  RotationStandardAxis=+Z  RotationAngle=0.0  RotationArbitraryAxis=[0 0 1]  FollAlignAxisA=+X  BaseAlignAxisA=+Y  FollAlignAxisB=+Y  BaseAlignAxisB=+Z  RotationSequenceAxes=FollowerAxes  RotationSequence=XYX  RotationSequenceAngles=[0 0 0]  RotationSequenceAnglesUnits=deg  RotationMatrix=[1 0 0; 0 1 0; 0 0 1]  Quaternion=[1 0 0 0]
  z-offset : sm_lib/Frames and Transforms/Rigid Transform  TranslationMethod=StandardAxis  TranslationStandardOffset=plane_offset  TranslationStandardOffsetUnits=m  TranslationStandardAxis=-Z  TranslationCartesianOffset=[0 0 0]  TranslationCartesianOffsetUnits=m  TranslationROffset=0  TranslationROffsetUnits=m  TranslationZOffset=0  TranslationZOffsetUnits=m  TranslationThetaOffset=0  TranslationThetaOffsetUnits=deg  RotationMethod=None  RotationAngleUnits=deg  RotationStandardAxis=+Z  RotationAngle=0.0  RotationArbitraryAxis=[0 0 1]  FollAlignAxisA=+X  BaseAlignAxisA=+Y  FollAlignAxisB=+Y  BaseAlignAxisB=+Z  RotationSequenceAxes=FollowerAxes  RotationSequence=XYX  RotationSequenceAngles=[0 0 0]  RotationSequenceAnglesUnits=deg  RotationMatrix=[1 0 0; 0 1 0; 0 0 1]  Quaternion=[1 0 0 0]
  Ground : PMIOPort  Side=Left
  "G " : PMIOPort  Port=2  Side=Left
  R : PMIOPort  Port=3  Side=Left
  connections:
  Brick Solid/LConn1 -- "G "/RConn1
  Brick Solid/RConn1 -- Ground/RConn1 -- z-offset/RConn1
  z-offset/LConn1 -- Translation/LConn1 -- R/RConn1
  Rotation/LConn1 -- Translation/RConn1
  Rotation/RConn1 -- Brick Solid1/RConn1

== system PhantomX_MK4/Motion Controller/Coordinator ==
  RL Observations : Inport
  Bus Selector : BusSelector  Commented=on  OutputSignals=Heights.Right Side Height.RBL Height,Heights.Right Side Height.RML Height,Heights.Right Side Height.RFL Height,Heights.Left Side Height.LBL Height,Heights.Left Side Height.LML Height,Heights.Left Side Height.LFL Height,x
  Constant12 : Constant  Value=[0 1]
  Demux : Demux  Commented=on  Outputs=8
  Derivative : Derivative  Commented=on
  Display : Display
  Display1 : Display
  Display2 : Display  Commented=on
  Mux : Mux  Commented=on  Inputs=7
  RL Agent : rllib/RL Agent  Commented=on  Agent=agentObj  ExternalActionAsInput=off  ProvideLastAction=off  ProvideCumRwd=off  TreatAsDirectFeedthrough=on  UseStrictObservationDataTypes=off
  Radians to Degrees : simulink_extras/Transformations/Radians to Degrees
  Reward Function : Subsystem  Commented=on
  Rotation Calculation : Custom_Library/Rotation Calculation  SystemSampleTime=-1  VariantActivationTime=update diagram  Latency=0  AutoFrameSizeCalculation=off
      settings: SourceProductName=Custom Hexapod Blocks
  Sine Wave : Sin  Frequency=(2*pi)/100  SampleTime=0
  Sine Wave1 : Sin  Frequency=(2*pi)/100  Phase=pi/2  SampleTime=0
  Tetrapod Gait : Subsystem  Commented=on
      settings: PortSchema="{\"entries\":[{\"content\":{\"sides\":[{\"content\":{\"connectorIds\":[\"Out6\",\"Out7\",\"Out8\"]},\"type\":\"ConnectorPlacement.EquallySpacedRectSide\",\"uuid\":\"8785c80f-3c92-41ee-ba1b-9daee48cf91e\"},{\"content\":{\"connectorIds\":[\"Out1\",\"Out2\",\"Out3\"],\"side\":\"RIGHT\"},\"type\":\"ConnectorPlacement.EquallySpacedRectSide\",\"uuid\":\"6c25dade-5a7d-4c01-9418-96963e8cfbe9\"},{\"content\":{\"connectorIds\":[\"Out4\",\"Out5\"],\"side\":\"TOP\"},\"type\":\"ConnectorPlacement.EquallySpacedRectSide\",\"uuid\":\"f808ef72-d784-4405-a2cb-8f4b4dbe6a2e\"}]},\"type\":\"ConnectorPlacement.EquallySpacedConnector\",\"uuid\":\"ab3b58c2-906e-4026-8eb1-165203241d6c\"}],\"packageUris\":[\"http://schema.mathworks.com/mf0/Connector/R2020b\"],\"version\":\"1.0\"}"
  Tripod Gait : Subsystem  Commented=on
      settings: PortSchema="{\"entries\":[{\"content\":{\"sides\":[{\"content\":{\"connectorIds\":[\"Out6\",\"Out7\",\"Out8\"]},\"type\":\"ConnectorPlacement.EquallySpacedRectSide\",\"uuid\":\"8785c80f-3c92-41ee-ba1b-9daee48cf91e\"},{\"content\":{\"connectorIds\":[\"Out1\",\"Out2\",\"Out3\"],\"side\":\"RIGHT\"},\"type\":\"ConnectorPlacement.EquallySpacedRectSide\",\"uuid\":\"6c25dade-5a7d-4c01-9418-96963e8cfbe9\"},{\"content\":{\"connectorIds\":[\"Out4\",\"Out5\"],\"side\":\"TOP\"},\"type\":\"ConnectorPlacement.EquallySpacedRectSide\",\"uuid\":\"f808ef72-d784-4405-a2cb-8f4b4dbe6a2e\"}]},\"type\":\"ConnectorPlacement.EquallySpacedConnector\",\"uuid\":\"ab3b58c2-906e-4026-8eb1-165203241d6c\"}],\"packageUris\":[\"http://schema.mathworks.com/mf0/Connector/R2020b\"],\"version\":\"1.0\"}"
  Tripod Gait1 : Subsystem
      settings: PortSchema="{\"entries\":[{\"content\":{\"sides\":[{\"content\":{\"connectorIds\":[\"Out6\",\"Out7\",\"Out8\"]},\"type\":\"ConnectorPlacement.EquallySpacedRectSide\",\"uuid\":\"8785c80f-3c92-41ee-ba1b-9daee48cf91e\"},{\"content\":{\"connectorIds\":[\"Out1\",\"Out2\",\"Out3\"],\"side\":\"RIGHT\"},\"type\":\"ConnectorPlacement.EquallySpacedRectSide\",\"uuid\":\"6c25dade-5a7d-4c01-9418-96963e8cfbe9\"},{\"content\":{\"connectorIds\":[\"Out4\",\"Out5\"],\"side\":\"TOP\"},\"type\":\"ConnectorPlacement.EquallySpacedRectSide\",\"uuid\":\"f808ef72-d784-4405-a2cb-8f4b4dbe6a2e\"}]},\"type\":\"ConnectorPlacement.EquallySpacedConnector\",\"uuid\":\"ab3b58c2-906e-4026-8eb1-165203241d6c\"}],\"packageUris\":[\"http://schema.mathworks.com/mf0/Connector/R2020b\"],\"version\":\"1.0\"}"
  Vector Concatenate : Concatenate
  Wave Gait : Subsystem  Commented=on
      settings: PortSchema="{\"entries\":[{\"content\":{\"sides\":[{\"content\":{\"connectorIds\":[\"Out6\",\"Out7\",\"Out8\"]},\"type\":\"ConnectorPlacement.EquallySpacedRectSide\",\"uuid\":\"8785c80f-3c92-41ee-ba1b-9daee48cf91e\"},{\"content\":{\"connectorIds\":[\"Out1\",\"Out2\",\"Out3\"],\"side\":\"RIGHT\"},\"type\":\"ConnectorPlacement.EquallySpacedRectSide\",\"uuid\":\"6c25dade-5a7d-4c01-9418-96963e8cfbe9\"},{\"content\":{\"connectorIds\":[\"Out4\",\"Out5\"],\"side\":\"TOP\"},\"type\":\"ConnectorPlacement.EquallySpacedRectSide\",\"uuid\":\"f808ef72-d784-4405-a2cb-8f4b4dbe6a2e\"}]},\"type\":\"ConnectorPlacement.EquallySpacedConnector\",\"uuid\":\"ab3b58c2-906e-4026-8eb1-165203241d6c\"}],\"packageUris\":[\"http://schema.mathworks.com/mf0/Connector/R2020b\"],\"version\":\"1.0\"}"
  Wave Gait1 : Subsystem  Commented=on
      settings: PortSchema="{\"entries\":[{\"content\":{\"sides\":[{\"content\":{\"connectorIds\":[\"Out6\",\"Out7\",\"Out8\"]},\"type\":\"ConnectorPlacement.EquallySpacedRectSide\",\"uuid\":\"8785c80f-3c92-41ee-ba1b-9daee48cf91e\"},{\"content\":{\"connectorIds\":[\"Out1\",\"Out2\",\"Out3\"],\"side\":\"RIGHT\"},\"type\":\"ConnectorPlacement.EquallySpacedRectSide\",\"uuid\":\"6c25dade-5a7d-4c01-9418-96963e8cfbe9\"},{\"content\":{\"connectorIds\":[\"Out4\",\"Out5\"],\"side\":\"TOP\"},\"type\":\"ConnectorPlacement.EquallySpacedRectSide\",\"uuid\":\"f808ef72-d784-4405-a2cb-8f4b4dbe6a2e\"}]},\"type\":\"ConnectorPlacement.EquallySpacedConnector\",\"uuid\":\"ab3b58c2-906e-4026-8eb1-165203241d6c\"}],\"packageUris\":[\"http://schema.mathworks.com/mf0/Connector/R2020b\"],\"version\":\"1.0\"}"
  RBL Offset : Outport
  RML Offset : Outport  Port=2
  RFL Offset : Outport  Port=3
  Rotation : Outport  Port=4
  Duty Cycle : Outport  Port=5
  Frequency : Outport  Port=6
  LBL Offset : Outport  Port=7
  LML Offset : Outport  Port=8
  LFL Offset : Outport  Port=9
  wires:
  Constant12/1 -> Rotation Calculation/1
  Rotation Calculation/1 -> Radians to Degrees/1, Rotation/1
  Radians to Degrees/1 -> Display/1
  Sine Wave/1 -> Vector Concatenate/1
  Sine Wave1/1 -> Vector Concatenate/2
  Vector Concatenate/1 -> Display1/1
  Demux/1 -> ?
  Demux/8 -> ?
  Demux/3 -> ?
  Bus Selector/7 -> Derivative/1  "<x>"
  Demux/6 -> ?
  Demux/4 -> ?
  Mux/1 -> RL Agent/1
  Bus Selector/1 -> Mux/1  "<RBL Height>"
  RL Observations/1 -> Bus Selector/1, Reward Function/1(RL Input)
  Reward Function/1(Reward) -> RL Agent/2
  Demux/7 -> ?
  Demux/5 -> ?
  Derivative/1 -> Mux/7
  Demux/2 -> ?
  RL Agent/1 -> Demux/1, Display2/1
  Bus Selector/5 -> Mux/5  "<LML Height>"
  Bus Selector/3 -> Mux/3  "<RFL Height>"
  Bus Selector/4 -> Mux/4  "<LBL Height>"
  Bus Selector/6 -> Mux/6  "<LFL Height>"
  Bus Selector/2 -> Mux/2  "<RML Height>"
  Wave Gait1/6(LBL Offset) -> ?
  Wave Gait1/8(LFL Offset) -> ?
  Wave Gait1/3(RFL Offset) -> ?
  Wave Gait1/1(RBL Offset) -> ?
  Wave Gait1/4(Frequency) -> ?
  Wave Gait1/5(Duty Cycle) -> ?
  Wave Gait1/7(LML Offset) -> ?
  Wave Gait1/2(RML Offset) -> ?
  Tripod Gait1/2(RML Offset) -> RML Offset/1
  Tripod Gait1/5(Duty Cycle) -> Duty Cycle/1
  Tripod Gait1/1(RBL Offset) -> RBL Offset/1
  Tripod Gait1/4(Frequency) -> Frequency/1
  Tripod Gait1/7(LML Offset) -> LML Offset/1
  Tripod Gait1/6(LBL Offset) -> LBL Offset/1
  Tripod Gait1/8(LFL Offset) -> LFL Offset/1
  Tripod Gait1/3(RFL Offset) -> RFL Offset/1
